simulink model "ISController"  (R2018a)
settings: Solver=FixedStepDiscrete  StartTime=0.0  StopTime=12  FixedStep=0.001  RelTol=1e-3  EnableMultiTasking=on
values from neighbouring files (symbols this model uses):
  Bx_ash_f = 11.7    [ISData.m]    (also in pacjeka_params.m)
  Bx_ash_r = 11.1    [ISData.m]    (also in pacjeka_params.m)
  Bx_snow_f = 10.2    [ISData.m]    (also in pacjeka_params.m)
  Bx_snow_r = 9.71    [ISData.m]    (also in pacjeka_params.m)
  By_ash_f = 8.86    [ISData.m]    (also in pacjeka_params.m)
  By_ash_r = 9.30    (= 9.3)    [ISData.m]    (also in pacjeka_params.m)
  By_snow_f = 19.1    [ISData.m]    (also in pacjeka_params.m)
  By_snow_r = 20.0    (= 20)    [ISData.m]    (also in pacjeka_params.m)
  Cx_ash_f = 1.69    [ISData.m]    (also in pacjeka_params.m)
  Cx_ash_r = 1.69    [ISData.m]    (also in pacjeka_params.m)
  Cx_snow_f = 1.96    [ISData.m]    (also in pacjeka_params.m)
  Cx_snow_r = 1.96    [ISData.m]    (also in pacjeka_params.m)
  Cy_ash_f = 1.19    [ISData.m]    (also in pacjeka_params.m)
  Cy_ash_r = 1.19    [ISData.m]    (also in pacjeka_params.m)
  Cy_snow_f = 0.550    (= 0.55)    [ISData.m]    (also in pacjeka_params.m)
  Cy_snow_r = 0.550    (= 0.55)    [ISData.m]    (also in pacjeka_params.m)
  D_phi = 16000    [ISData.m]    (also in IS_2impulse.m; IS_3impulse.m; IS_4impulse.m; InputShaper.m)
  D_theta = 30960    [ISData.m]    (also in IS_2impulse.m; IS_3impulse.m; IS_4impulse.m; InputShaper.m)
  delta_r = 0    [ISData.m]    (also in IS_2impulse.m; IS_3impulse.m; IS_4impulse.m; InputShaper.m)
  DLCTest = [0 0 0 0 0 0 0 0 0 0 0 0 ... (12003 elements, 12003x1)]    [DLCTest.mat]
  epsilon = 0.4    [ISData.m]    (also in IS_2impulse.m; IS_3impulse.m; IS_4impulse.m; InputShaper.m)
  Ex_ash_f = 0.377    [ISData.m]    (also in pacjeka_params.m)
  Ex_ash_r = 0.362    [ISData.m]    (also in pacjeka_params.m)
  Ex_snow_f = 0.651    [ISData.m]    (also in pacjeka_params.m)
  Ex_snow_r = 0.624    [ISData.m]    (also in pacjeka_params.m)
  Ey_ash_f = -1.21    [ISData.m]    (also in pacjeka_params.m)
  Ey_ash_r = -1.11    [ISData.m]    (also in pacjeka_params.m)
  Ey_snow_f = -2.1    [ISData.m]    (also in pacjeka_params.m)
  Ey_snow_r = -1.93    [ISData.m]    (also in pacjeka_params.m)
  g = 9.81    [ISData.m]    (also in IS_2impulse.m; IS_3impulse.m; IS_4impulse.m; InputShaper.m)
  h = 0.5    [ISData.m]    (also in IS_2impulse.m; IS_3impulse.m; IS_4impulse.m; InputShaper.m)
  Iw = 4    [ISData.m]    (also in IS_2impulse.m; IS_3impulse.m; IS_4impulse.m; InputShaper.m)
  Ixx = 602.1923    [ISData.m]    (also in IS_2impulse.m; IS_3impulse.m; IS_4impulse.m; InputShaper.m)
  Iyy = 2.7370e+03    (= 2737)    [ISData.m]    (also in IS_2impulse.m; IS_3impulse.m; IS_4impulse.m; InputShaper.m)
  Izz = 3070    [ISData.m]    (also in IS_2impulse.m; IS_3impulse.m; IS_4impulse.m; InputShaper.m)
  K_phi = 178000    [ISData.m]    (also in IS_2impulse.m; IS_3impulse.m; IS_4impulse.m; InputShaper.m)
  K_theta = 363540    [ISData.m]    (also in IS_2impulse.m; IS_3impulse.m; IS_4impulse.m; InputShaper.m)
  l_f = 1.2110    (= 1.211)    [ISData.m]    (also in IS_2impulse.m; IS_3impulse.m; IS_4impulse.m; InputShaper.m)
  l_r = 1.4590    (= 1.459)    [ISData.m]    (also in IS_2impulse.m; IS_3impulse.m; IS_4impulse.m; InputShaper.m)
  m = 1830    [ISData.m]    (also in IS_2impulse.m; IS_3impulse.m; IS_4impulse.m; InputShaper.m)
  mu_x_ash_f = 1.20    (= 1.2)    [ISData.m]    (also in pacjeka_params.m)
  mu_x_ash_r = 1.20    (= 1.2)    [ISData.m]    (also in pacjeka_params.m)
  mu_x_snow_f = 0.407    [ISData.m]    (also in pacjeka_params.m)
  mu_x_snow_r = 0.409    [ISData.m]    (also in pacjeka_params.m)
  mu_y_ash_f = 0.935    [ISData.m]    (also in pacjeka_params.m)
  mu_y_ash_r = 0.961    [ISData.m]    (also in pacjeka_params.m)
  mu_y_snow_f = 0.383    [ISData.m]    (also in pacjeka_params.m)
  mu_y_snow_r = 0.394    [ISData.m]    (also in pacjeka_params.m)
  omega0 = Vx0/Rw    (= 64.7813411079)    [ISData.m]    (also in IS_2impulse.m = 74.1; IS_3impulse.m = 74.1; IS_4impulse.m = 74.1; InputShaper.m = 74.0666666667)
  road = 1    [ISData.m]    (also in IS_2impulse.m; IS_3impulse.m; IS_4impulse.m; InputShaper.m)
  Rw = 0.3430    (= 0.343)    [ISData.m]    (also in IS_2impulse.m = 0.3; IS_3impulse.m = 0.3; IS_4impulse.m = 0.3; InputShaper.m = 0.3)
  thetaSW_actual = [thetaSW_actual, deltaSW]    [IS_2impulse.m]    (also in InputShaper.m; InputShaper2.m; thetaSW_IS_L.mat = [0 0 0 0 0 0 0 0 0 0 0 0 ... (12003 elements, 1x12003)]; thetaSW_IS_NL.mat = [0 0 0 0 0 0 0 0 0 0 0 0 ... (12003 elements, 1x12003)])
  Ts = 0.001    [ISData.m]    (also in IS_2impulse.m; IS_3impulse.m; IS_4impulse.m; InputShaper.m)
  Tsmall = 0.001    [ISData.m]    (also in IS_2impulse.m; IS_3impulse.m; IS_4impulse.m; InputShaper.m)
  Vx0 = 22.22    [ISData.m]    (also in IS_2impulse.m = states(3); IS_3impulse.m = states(3); IS_4impulse.m = states(3); InputShaper.m = states(3))
  w = 0.7700    (= 0.77)    [ISData.m]    (also in IS_2impulse.m; IS_3impulse.m; IS_4impulse.m; InputShaper.m)
libraries: simulink x2
(part 2 of 4)

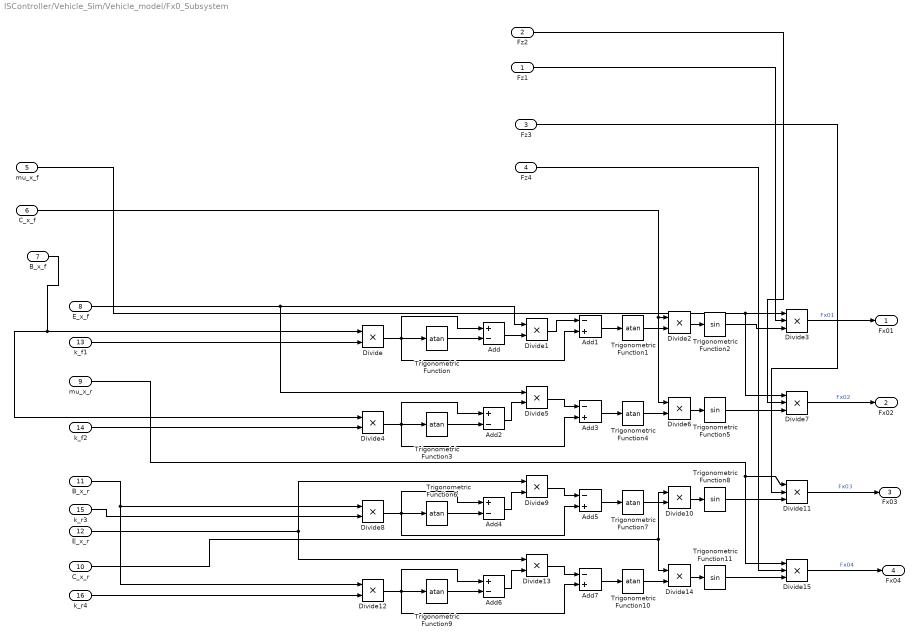
== system ISController/Vehicle_Sim/Vehicle_model/Fx0_Subsystem ==
  Fz1 : Inport  OutDataTypeStr=double  SampleTime=Ts
  Fz2 : Inport  Port=2  OutDataTypeStr=double  SampleTime=Ts
  Fz3 : Inport  Port=3  OutDataTypeStr=double  SampleTime=Ts
  Fz4 : Inport  Port=4  OutDataTypeStr=double  SampleTime=Ts
  mu_x_f : Inport  Port=5
  C_x_f : Inport  Port=6
  B_x_f : Inport  Port=7
  E_x_f : Inport  Port=8
  mu_x_r : Inport  Port=9
  C_x_r : Inport  Port=10
  B_x_r : Inport  Port=11
  E_x_r : Inport  Port=12
  k_f1 : Inport  Port=13
  k_f2 : Inport  Port=14
  k_r3 : Inport  Port=15
  k_r4 : Inport  Port=16
  Add{,2,4,6} (4 alike) : Sum  Inputs=+-
  Add{1,3,5,7} (4 alike) : Sum  Inputs=-+
  Divide{,1..2,4..6,8..10,12..14} (12 alike) : Product  Inputs=**
  Divide{3,7,11,15} (4 alike) : Product  Inputs=***
  Trigonometric Function{,1,3..4,6..7,9..10} (8 alike) : Trigonometry  Operator=atan
  Trigonometric Function{2,5,8,11} (4 alike) : Trigonometry
  Fx01 : Outport  OutDataTypeStr=double  SampleTime=Ts
  Fx02 : Outport  Port=2  OutDataTypeStr=double  SampleTime=Ts
  Fx03 : Outport  Port=3  OutDataTypeStr=double  SampleTime=Ts
  Fx04 : Outport  Port=4  OutDataTypeStr=double  SampleTime=Ts
  wires:
  Divide13/1 -> Add7/1
  Trigonometric Function2/1 -> Divide3/3
  Divide11/1 -> Fx03/1  "Fx03"
  Divide7/1 -> Fx02/1  "Fx02"
  Divide1/1 -> Add1/1
  Trigonometric Function/1 -> Add/2
  Divide15/1 -> Fx04/1  "Fx04"
  Add/1 -> Divide1/2
  Divide/1 -> Add1/2, Add/1, Trigonometric Function/1
  k_f1/1 -> Divide/2
  k_r4/1 -> Divide12/2
  k_r3/1 -> Divide8/2
  Divide6/1 -> Trigonometric Function5/1
  Divide4/1 -> Add3/2, Add2/1, Trigonometric Function3/1
  Divide5/1 -> Add3/1
  Trigonometric Function3/1 -> Add2/2
  Add2/1 -> Divide5/2
  E_x_f/1 -> Divide5/1, Divide1/1
  B_x_f/1 -> Divide4/1, Divide/1
  Trigonometric Function4/1 -> Divide6/2
  C_x_f/1 -> Divide6/1, Divide2/1
  Trigonometric Function5/1 -> Divide7/3
  Add3/1 -> Trigonometric Function4/1
  C_x_r/1 -> Divide14/1, Divide10/1
  B_x_r/1 -> Divide12/1, Divide8/1
  E_x_r/1 -> Divide9/1, Divide13/1
  mu_x_r/1 -> Divide15/1, Divide11/1
  Fz2/1 -> Divide7/2
  mu_x_f/1 -> Divide7/1, Divide3/1
  k_f2/1 -> Divide4/2
  Fz1/1 -> Divide3/2
  Fz3/1 -> Divide11/2
  Add1/1 -> Trigonometric Function1/1
  Add4/1 -> Divide9/2
  Divide8/1 -> Add5/2, Add4/1, Trigonometric Function6/1
  Trigonometric Function8/1 -> Divide11/3
  Add5/1 -> Trigonometric Function7/1
  Trigonometric Function6/1 -> Add4/2
  Divide10/1 -> Trigonometric Function8/1
  Trigonometric Function7/1 -> Divide10/2
  Fz4/1 -> Divide15/2
  Divide9/1 -> Add5/1
  Trigonometric Function1/1 -> Divide2/2
  Divide3/1 -> Fx01/1  "Fx01"
  Divide2/1 -> Trigonometric Function2/1
  Trigonometric Function10/1 -> Divide14/2
  Trigonometric Function9/1 -> Add6/2
  Divide14/1 -> Trigonometric Function11/1
  Divide12/1 -> Add7/2, Add6/1, Trigonometric Function9/1
  Trigonometric Function11/1 -> Divide15/3
  Add7/1 -> Trigonometric Function10/1
  Add6/1 -> Divide13/2

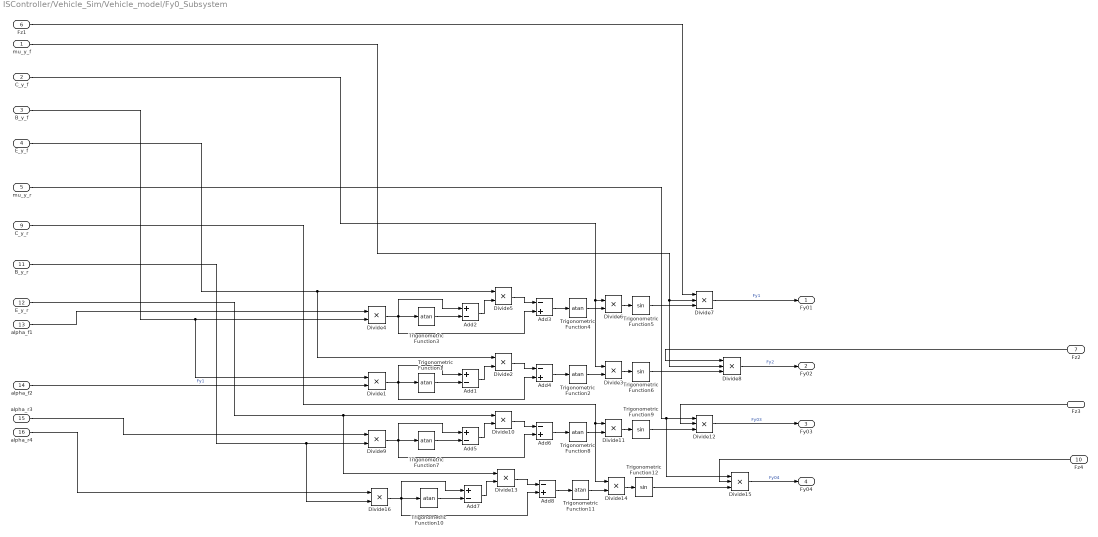
== system ISController/Vehicle_Sim/Vehicle_model/Fy0_Subsystem ==
  mu_y_f : Inport  OutDataTypeStr=double  SampleTime=Ts
  C_y_f : Inport  Port=2  OutDataTypeStr=double  SampleTime=Ts
  B_y_f : Inport  Port=3  OutDataTypeStr=double  SampleTime=Ts
  E_y_f : Inport  Port=4  OutDataTypeStr=double  SampleTime=Ts
  mu_y_r : Inport  Port=5  OutDataTypeStr=double  SampleTime=Ts
  Fz1 : Inport  Port=6  OutDataTypeStr=double  SampleTime=Ts
  Fz2 : Inport  Port=7  OutDataTypeStr=double  SampleTime=Ts
  Fz3 : Inport  Port=8  OutDataTypeStr=double  SampleTime=Ts
  C_y_r : Inport  Port=9  OutDataTypeStr=double  SampleTime=Ts
  Fz4 : Inport  Port=10  OutDataTypeStr=double  SampleTime=Ts
  B_y_r : Inport  Port=11  OutDataTypeStr=double  SampleTime=Ts
  E_y_r : Inport  Port=12  OutDataTypeStr=double  SampleTime=Ts
  alpha_f1 : Inport  Port=13  OutDataTypeStr=double  SampleTime=Ts
  alpha_f2 : Inport  Port=14  OutDataTypeStr=double  SampleTime=Ts
  alpha_r3 : Inport  Port=15  OutDataTypeStr=double  SampleTime=Ts
  alpha_r4 : Inport  Port=16  OutDataTypeStr=double  SampleTime=Ts
  Add{1..2,5,7} (4 alike) : Sum  Inputs=+-
  Add{3..4,6,8} (4 alike) : Sum  Inputs=-+
  Divide{1..6,9..11,13..14,16} (12 alike) : Product  Inputs=**
  Divide{7..8,12,15} (4 alike) : Product  Inputs=***
  Trigonometric Function{1..4,7..8,10..11} (8 alike) : Trigonometry  Operator=atan
  Trigonometric Function{5..6,9,12} (4 alike) : Trigonometry
  Fy01 : Outport  OutDataTypeStr=double  SampleTime=Ts
  Fy02 : Outport  Port=2  OutDataTypeStr=double  SampleTime=Ts
  Fy03 : Outport  Port=3  OutDataTypeStr=double  SampleTime=Ts
  Fy04 : Outport  Port=4  OutDataTypeStr=double  SampleTime=Ts
  wires:
  Add6/1 -> Trigonometric Function8/1
  Trigonometric Function9/1 -> Divide12/3
  alpha_r3/1 -> Divide9/1
  alpha_r4/1 -> Divide16/1
  C_y_f/1 -> Divide6/1, Divide3/1
  B_y_f/1 -> Divide4/2, Divide1/1
  alpha_f1/1 -> Divide4/1
  E_y_r/1 -> Divide13/1, Divide10/1
  B_y_r/1 -> Divide16/2, Divide9/2
  mu_y_r/1 -> Divide12/1, Divide15/1
  E_y_f/1 -> Divide5/1, Divide2/1
  mu_y_f/1 -> Divide8/2, Divide7/2
  Trigonometric Function1/1 -> Add1/2
  Add1/1 -> Divide2/2
  Trigonometric Function6/1 -> Divide8/3
  Trigonometric Function2/1 -> Divide3/2
  Divide1/1 -> Add4/2, Add1/1, Trigonometric Function1/1
  Divide3/1 -> Trigonometric Function6/1
  Divide2/1 -> Add4/1
  Add4/1 -> Trigonometric Function2/1
  Fz4/1 -> Divide15/2
  Fz3/1 -> Divide12/2
  Fz2/1 -> Divide8/1
  Fz1/1 -> Divide7/1
  C_y_r/1 -> Divide14/1, Divide11/1
  Divide15/1 -> Fy04/1  "Fy04"
  Trigonometric Function12/1 -> Divide15/3
  Add8/1 -> Trigonometric Function11/1
  Divide16/1 -> Add8/2, Add7/1, Trigonometric Function10/1
  Trigonometric Function11/1 -> Divide14/2
  Add7/1 -> Divide13/2
  Divide13/1 -> Add8/1
  Divide14/1 -> Trigonometric Function12/1
  Trigonometric Function10/1 -> Add7/2
  Divide12/1 -> Fy03/1  "Fy03"
  Divide9/1 -> Add6/2, Add5/1, Trigonometric Function7/1
  Trigonometric Function7/1 -> Add5/2
  Add5/1 -> Divide10/2
  Trigonometric Function5/1 -> Divide7/3
  Divide11/1 -> Trigonometric Function9/1
  Divide6/1 -> Trigonometric Function5/1
  Add3/1 -> Trigonometric Function4/1
  Trigonometric Function3/1 -> Add2/2
  Divide10/1 -> Add6/1
  Add2/1 -> Divide5/2
  Trigonometric Function4/1 -> Divide6/2
  Divide4/1 -> Add3/2, Add2/1, Trigonometric Function3/1
  Divide5/1 -> Add3/1
  Trigonometric Function8/1 -> Divide11/2
  Divide7/1 -> Fy01/1  "Fy1"
  Divide8/1 -> Fy02/1  "Fy2"
  alpha_f2/1 -> Divide1/2  "Fy1"

== system ISController/Vehicle_Sim/Vehicle_model/Fy0_to_Fy_subsystem ==
  mu_x_f : Inport  OutDataTypeStr=double  SampleTime=Ts
  mu_x_r : Inport  Port=2  OutDataTypeStr=double  SampleTime=Ts
  Fx01 : Inport  Port=3  OutDataTypeStr=double  SampleTime=Ts
  Fx02 : Inport  Port=4  OutDataTypeStr=double  SampleTime=Ts
  Fx03 : Inport  Port=5  OutDataTypeStr=double  SampleTime=Ts
  Fx04 : Inport  Port=6  OutDataTypeStr=double  SampleTime=Ts
  Fz1 : Inport  Port=7  OutDataTypeStr=double  SampleTime=Ts
  Fz2 : Inport  Port=8  OutDataTypeStr=double  SampleTime=Ts
  Fz3 : Inport  Port=9  OutDataTypeStr=double  SampleTime=Ts
  Fz4 : Inport  Port=10  OutDataTypeStr=double  SampleTime=Ts
  Fy01 : Inport  Port=11  OutDataTypeStr=double  SampleTime=Ts
  Fy02 : Inport  Port=12  OutDataTypeStr=double  SampleTime=Ts
  Fy03 : Inport  Port=13  OutDataTypeStr=double  SampleTime=Ts
  Fy04 : Inport  Port=14  OutDataTypeStr=double  SampleTime=Ts
  Add{,1..3} (4 alike) : Sum  Inputs=+-
  Constant{,1..3} (4 alike) : Constant
  Divide{,3,6,9} (4 alike) : Product  Inputs=*/
  Divide{1..2,4..5,7..8,10..11} (8 alike) : Product  Inputs=**
  Sqrt{,1..3} (4 alike) : Sqrt  SaturateOnIntegerOverflow=on
  Square{,1..3} (4 alike) : Math  Operator=square  RndMeth=Zero  SaturateOnIntegerOverflow=on
  local_Fy1 : Outport  OutDataTypeStr=double  SampleTime=Ts
  local_Fy2 : Outport  Port=2  OutDataTypeStr=double  SampleTime=Ts
  local_Fy3 : Outport  Port=3  OutDataTypeStr=double  SampleTime=Ts
  lcoal_Fy4 : Outport  Port=4  OutDataTypeStr=double  SampleTime=Ts
  wires:
  Divide1/1 -> Divide/2
  Divide/1 -> Square/1
  Constant/1 -> Add/1
  Divide2/1 -> local_Fy1/1  "Fy1"
  Divide11/1 -> lcoal_Fy4/1  "Fy4"
  Fz4/1 -> Divide10/2  "Fz4"
  mu_x_f/1 -> Divide4/1, Divide1/1  "mu_x_f"
  Fx04/1 -> Divide9/1  "Fx04"
  Fx01/1 -> Divide/1  "Fx01"
  Fz3/1 -> Divide7/2  "Fz3"
  Fx02/1 -> Divide3/1  "Fx02"
  mu_x_r/1 -> Divide10/1, Divide7/1  "mu_x_r"
  Fx03/1 -> Divide6/1  "Fx03"
  Fz1/1 -> Divide1/2  "Fz1"
  Fz2/1 -> Divide4/2  "Fz2"
  Square2/1 -> Add2/2
  Divide6/1 -> Square2/1
  Sqrt2/1 -> Divide8/1
  Constant2/1 -> Add2/1
  Sqrt3/1 -> Divide11/1
  Constant3/1 -> Add3/1
  Add3/1 -> Sqrt3/1
  Divide9/1 -> Square3/1
  Square3/1 -> Add3/2
  Add/1 -> Sqrt/1
  Square/1 -> Add/2
  Divide10/1 -> Divide9/2
  Divide8/1 -> local_Fy3/1  "Fy3"
  Sqrt/1 -> Divide2/1
  Divide4/1 -> Divide3/2
  Square1/1 -> Add1/2
  Divide3/1 -> Square1/1
  Constant1/1 -> Add1/1
  Fy02/1 -> Divide5/2  "Fy02"
  Add1/1 -> Sqrt1/1
  Sqrt1/1 -> Divide5/1
  Divide7/1 -> Divide6/2
  Add2/1 -> Sqrt2/1
  Fy03/1 -> Divide8/2  "Fy03"
  Divide5/1 -> local_Fy2/1  "Fy2"
  Fy01/1 -> Divide2/2  "Fy01"
  Fy04/1 -> Divide11/2  "Fy04"

== system ISController/Vehicle_Sim/Vehicle_model/Fz_Subsystem ==
  l_f : Inport  OutDataTypeStr=double  SampleTime=Ts
  l_r : Inport  Port=2  OutDataTypeStr=double  SampleTime=Ts
  k_phi : Inport  Port=3  OutDataTypeStr=double  SampleTime=Ts
  d_phi : Inport  Port=4  OutDataTypeStr=double  SampleTime=Ts
  theta_dot : Inport  Port=5  OutDataTypeStr=double  SampleTime=Ts
  theta : Inport  Port=6  OutDataTypeStr=double  SampleTime=Ts
  phi_dot : Inport  Port=7  OutDataTypeStr=double  SampleTime=Ts
  phi : Inport  Port=8  OutDataTypeStr=double  SampleTime=Ts
  K_theta : Inport  Port=9  OutDataTypeStr=double  SampleTime=Ts
  D_theta : Inport  Port=10  OutDataTypeStr=double  SampleTime=Ts
  w : Inport  Port=11  OutDataTypeStr=double  SampleTime=Ts
  Add{,1,3..4,6} (5 alike) : Sum
  Add2 : Sum  Inputs=+-+
  Add5 : Sum  Inputs=--
  Add7 : Sum  Inputs=-+
  Add8 : Sum  Inputs=-+
  Divide{,1..2,5} (4 alike) : Product  Inputs=*/
  Divide3 : Product  Inputs=**
  Divide4 : Product  Inputs=**
  Gain : Gain  Gain=-1  OutDataTypeStr=double
  Gain1 : Gain  Gain=0.5
  mg : Constant  Value=m*g
  tau_phi_subsystem : Subsystem
  tau_theta_subsystem : Subsystem
  Fz1 : Outport  OutDataTypeStr=double  SampleTime=Ts
  Fz2 : Outport  Port=2  OutDataTypeStr=double  SampleTime=Ts
  Fz3 : Outport  Port=3  OutDataTypeStr=double  SampleTime=Ts
  Fz4 : Outport  Port=4  OutDataTypeStr=double  SampleTime=Ts
  wires:
  phi/1 -> tau_phi_subsystem/4(phi)
  theta/1 -> tau_theta_subsystem/2(theta)
  phi_dot/1 -> tau_phi_subsystem/3(phi_dot)
  w/1 -> Divide2/2, Gain/1
  Add1/1 -> Divide2/1
  Divide2/1 -> Add3/1
  Add2/1 -> Divide5/1
  d_phi/1 -> tau_phi_subsystem/2(D_phi)
  D_theta/1 -> tau_theta_subsystem/4(D_theta)
  l_r/1 -> Divide4/1, Add5/1
  theta_dot/1 -> tau_theta_subsystem/1(theta_dot)
  tau_theta_subsystem/1(tau_theta) -> Add2/1  "tau_theta"
  K_theta/1 -> tau_theta_subsystem/3(K_theta)
  Add8/1 -> Fz1/1  "Fz1"
  Add/1 -> Add8/2, Add4/1  "E1"
  Divide3/1 -> Add2/2
  Divide5/1 -> Fz4/1, Add8/1, Add7/1, Add6/1  "Fz4"
  Add3/1 -> Gain1/1
  Add5/1 -> Divide5/2
  Gain1/1 -> Add7/2, Add4/2, Add/2  "E2"
  Add4/1 -> Divide3/2
  Add6/1 -> Fz3/1  "Fz3"
  Divide/1 -> Divide4/2, Add6/2  "E3"
  mg/1 -> Add3/2
  Divide4/1 -> Add2/3
  Divide1/1 -> Add/1
  k_phi/1 -> tau_phi_subsystem/1(K_phi)
  l_f/1 -> Add5/2, Divide3/1
  Add7/1 -> Fz2/1  "Fz2"
  tau_phi_subsystem/1(tau_phi_f) -> Divide1/1, Add1/1  "tau_phi_f"
  tau_phi_subsystem/2(tau_phi_r) -> Add1/2, Divide/1  "tau_phi_r"
  Gain/1 -> Divide1/2, Divide/2

== system ISController/Vehicle_Sim/Vehicle_model/Pacjeka_parameters_Subsystem ==
  surface_condition : Inport  OutDataTypeStr=double  SampleTime=Ts
  Ashphalt_condition_subsystem : Subsystem  TreatAsAtomicUnit=on
  Demux : Demux  Outputs=2
  If : If  IfExpression=(u1==1)
  Merge : Merge
  Snow_condition_subsystem : Subsystem  TreatAsAtomicUnit=on
  front : Outport  OutDataTypeStr=double  SampleTime=Ts
  rear : Outport  Port=2  OutDataTypeStr=double  SampleTime=Ts
  wires:
  Demux/2 -> rear/1  "rear"
  Merge/1 -> Demux/1
  If/1 -> Ashphalt_condition_subsystem/Action
  If/2 -> Snow_condition_subsystem/Action
  Demux/1 -> front/1  "front"
  surface_condition/1 -> If/1
  Ashphalt_condition_subsystem/1(Out1) -> Merge/1
  Snow_condition_subsystem/1(Out1) -> Merge/2

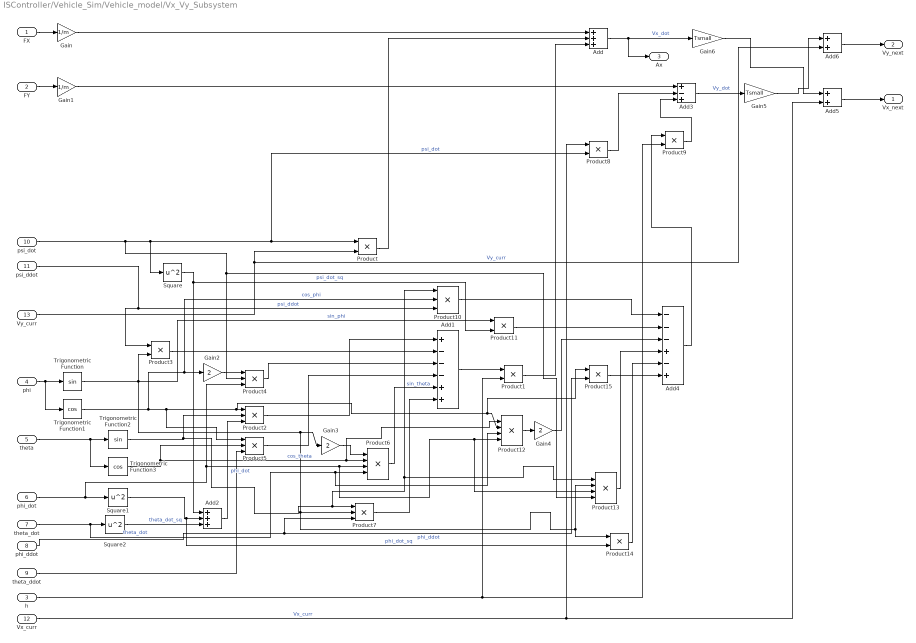
== system ISController/Vehicle_Sim/Vehicle_model/Vx_Vy_Subsystem ==
  FX : Inport  OutDataTypeStr=double  SampleTime=Ts
  FY : Inport  Port=2  OutDataTypeStr=double  SampleTime=Ts
  h : Inport  Port=3  OutDataTypeStr=double  SampleTime=Ts
  phi : Inport  Port=4  OutDataTypeStr=double  SampleTime=Ts
  theta : Inport  Port=5  OutDataTypeStr=double  SampleTime=Ts
  phi_dot : Inport  Port=6  OutDataTypeStr=double  SampleTime=Ts
  theta_dot : Inport  Port=7  OutDataTypeStr=double  SampleTime=Ts
  phi_ddot : Inport  Port=8  OutDataTypeStr=double  SampleTime=Ts
  theta_ddot : Inport  Port=9  OutDataTypeStr=double  SampleTime=Ts
  psi_dot : Inport  Port=10  OutDataTypeStr=double  SampleTime=Ts
  psi_ddot : Inport  Port=11  OutDataTypeStr=double  SampleTime=Ts
  Vx_curr : Inport  Port=12  OutDataTypeStr=double  SampleTime=Tsmall
  Vy_curr : Inport  Port=13  OutDataTypeStr=double  SampleTime=Tsmall
  Add : Sum  Inputs=+++
  Add1 : Sum  Inputs=+---++
  Add2 : Sum  Inputs=+++
  Add3 : Sum  Inputs=+-+
  Add4 : Sum  Inputs=---+-+
  Add5 : Sum
  Add6 : Sum
  Gain : Gain  Gain=1/m
  Gain1 : Gain  Gain=1/m
  Gain2 : Gain  Gain=2
  Gain3 : Gain  Gain=2
  Gain4 : Gain  Gain=2
  Gain5 : Gain  Gain=Tsmall
  Gain6 : Gain  Gain=Tsmall
  Product{,1,3,8..9,11,14..15} (8 alike) : Product
  Product{2,4..5,7,10} (5 alike) : Product  Inputs=3
  Product12 : Product  Inputs=4
  Product13 : Product  Inputs=4
  Product6 : Product  Inputs=4
  Square : Math  Operator=square  RndMeth=Zero  SaturateOnIntegerOverflow=on
  Square1 : Math  Operator=square  RndMeth=Zero  SaturateOnIntegerOverflow=on
  Square2 : Math  Operator=square  RndMeth=Zero  SaturateOnIntegerOverflow=on
  Trigonometric Function : Trigonometry
  Trigonometric Function1 : Trigonometry  Operator=cos
  Trigonometric Function2 : Trigonometry
  Trigonometric Function3 : Trigonometry  Operator=cos
  Vx_next : Outport  OutDataTypeStr=double  SampleTime=Tsmall
  Vy_next : Outport  Port=2  OutDataTypeStr=double  SampleTime=Tsmall
  Ax : Outport  Port=3
  wires:
  FX/1 -> Gain/1
  FY/1 -> Gain1/1
  Gain/1 -> Add/1
  psi_dot/1 -> Product4/2, Product13/4, Square/1, Product8/2, Product/1  "psi_dot"
  Product/1 -> Add/2
  Vy_curr/1 -> Add6/2, Product/2  "Vy_curr"
  Product1/1 -> Add/3
  phi/1 -> Trigonometric Function1/1, Trigonometric Function/1
  theta/1 -> Trigonometric Function3/1, Trigonometric Function2/1
  Add1/1 -> Product1/1
  h/1 -> Product9/2, Product1/2
  Add2/1 -> Product2/3
  Square/1 -> Product11/2, Add2/1  "psi_dot_sq"
  Square1/1 -> Product14/2, Add2/2  "phi_dot_sq"
  phi_dot/1 -> Product13/3, Product12/4, Product6/3, Product4/3, Square1/1  "phi_dot"
  Square2/1 -> Add2/3  "theta_dot_sq"
  theta_dot/1 -> Product12/3, Product6/4, Square2/1  "theta_dot"
  Product2/1 -> Add1/1
  Trigonometric Function/1 -> Product11/1, Product14/1, Product13/2, Product7/2, Gain3/1, Product3/2  "sin_phi"
  psi_ddot/1 -> Product10/3, Product3/1  "psi_ddot"
  Product3/1 -> Add1/2
  Gain2/1 -> Product4/1
  Product4/1 -> Add1/3
  Trigonometric Function3/1 -> Product5/2, Product12/1, Product6/2  "cos_theta"
  theta_ddot/1 -> Product5/3
  Product5/1 -> Add1/4
  Product6/1 -> Add1/5
  Gain3/1 -> Product6/1
  phi_ddot/1 -> Product15/2, Product7/3  "phi_ddot"
  Product7/1 -> Add1/6
  Add/1 -> Ax/1, Gain6/1  "Vx_dot"
  Gain1/1 -> Add3/1
  Vx_curr/1 -> Add5/2, Product8/1  "Vx_curr"
  Product8/1 -> Add3/2
  Add4/1 -> Product9/1
  Product9/1 -> Add3/3
  Product10/1 -> Add4/1
  Trigonometric Function2/1 -> Product13/1, Product10/1, Product7/1, Product2/2  "sin_theta"
  Trigonometric Function1/1 -> Product10/2, Gain2/1, Product5/1, Product15/1, Product12/2, Product2/1  "cos_phi"
  Product11/1 -> Add4/2
  Product12/1 -> Gain4/1
  Gain4/1 -> Add4/3
  Product13/1 -> Add4/4
  Product14/1 -> Add4/5
  Product15/1 -> Add4/6
  Add3/1 -> Gain5/1  "Vy_dot"
  Gain5/1 -> Add6/1
  Add5/1 -> Vx_next/1
  Gain6/1 -> Add5/1
  Add6/1 -> Vy_next/1

== system ISController/Vehicle_Sim/Vehicle_model/local_to_global_Fx_Fy_Subsystem ==
  local_Fx1 : Inport  OutDataTypeStr=double  SampleTime=Ts
  local_Fx2 : Inport  Port=2  OutDataTypeStr=double  SampleTime=Ts
  local_Fx3 : Inport  Port=3  OutDataTypeStr=double  SampleTime=Ts
  local_Fx4 : Inport  Port=4  OutDataTypeStr=double  SampleTime=Ts
  local_Fy1 : Inport  Port=5  OutDataTypeStr=double  SampleTime=Ts
  local_Fy2 : Inport  Port=6  OutDataTypeStr=double  SampleTime=Ts
  local_Fy3 : Inport  Port=7  OutDataTypeStr=double  SampleTime=Ts
  local_Fy4 : Inport  Port=8  OutDataTypeStr=double  SampleTime=Ts
  delta_f2 : Inport  Port=9  OutDataTypeStr=double  SampleTime=Ts
  Add{,1..3} (4 alike) : Sum
  Constant : Constant  Value=delta_r
  Cos : Trigonometry  Operator=cos
  Cos1 : Trigonometry  Operator=cos
  Product{,1..15} (16 alike) : Product
  Sin : Trigonometry
  Sin1 : Trigonometry
  Subtract{,1..3} (4 alike) : Sum  Inputs=+-
  Fx1 : Outport  OutDataTypeStr=double  SampleTime=Ts
  Fx2 : Outport  Port=2  OutDataTypeStr=double  SampleTime=Ts
  Fx3 : Outport  Port=3  OutDataTypeStr=double  SampleTime=Ts
  Fx4 : Outport  Port=4  OutDataTypeStr=double  SampleTime=Ts
  Fy1 : Outport  Port=5  OutDataTypeStr=double  SampleTime=Ts
  Fy2 : Outport  Port=6  OutDataTypeStr=double  SampleTime=Ts
  Fy3 : Outport  Port=7  OutDataTypeStr=double  SampleTime=Ts
  Fy4 : Outport  Port=8  OutDataTypeStr=double  SampleTime=Ts
  wires:
  delta_f2/1 -> Cos/1, Sin/1
  local_Fx1/1 -> Product2/2, Product/1  "local_Fx1"
  local_Fx2/1 -> Product6/2, Product4/2  "local_Fx2"
  local_Fx3/1 -> Product10/2, Product8/1  "local_Fx3"
  local_Fx4/1 -> Product14/1, Product12/1  "local_Fx4"
  local_Fy1/1 -> Product3/2, Product1/1  "local_Fy1"
  local_Fy2/1 -> Product7/2, Product5/2  "local_Fy2"
  local_Fy3/1 -> Product11/2, Product9/2  "local_Fy3"
  local_Fy4/1 -> Product15/1, Product13/1  "local_Fy4"
  Cos/1 -> Product7/1, Product4/1, Product3/1, Product/2  "cosDeltaf2"
  Sin/1 -> Product5/1, Product6/1, Product2/1, Product1/2  "sinDeltaf2"
  Product/1 -> Subtract/1
  Product1/1 -> Subtract/2
  Subtract/1 -> Fx1/1  "Fx1"
  Product2/1 -> Add/1
  Product3/1 -> Add/2
  Add/1 -> Fy1/1  "Fy1"
  Product6/1 -> Add1/1
  Product7/1 -> Add1/2
  Product4/1 -> Subtract1/1
  Product5/1 -> Subtract1/2
  Subtract1/1 -> Fx2/1  "Fx2"
  Add1/1 -> Fy2/1  "Fy2"
  Constant/1 -> Cos1/1, Sin1/1
  Sin1/1 -> Product14/2, Product13/2, Product10/1, Product9/1  "sinDelta_r"
  Cos1/1 -> Product15/2, Product12/2, Product11/1, Product8/2  "cosDelta_r"
  Product8/1 -> Subtract2/1
  Product9/1 -> Subtract2/2
  Subtract2/1 -> Fx3/1  "Fx3"
  Product10/1 -> Add2/1
  Product11/1 -> Add2/2
  Add2/1 -> Fy3/1  "Fy3"
  Product12/1 -> Subtract3/1
  Product13/1 -> Subtract3/2
  Product14/1 -> Add3/1
  Product15/1 -> Add3/2
  Subtract3/1 -> Fx4/1  "Fx4"
  Add3/1 -> Fy4/1  "Fy4"

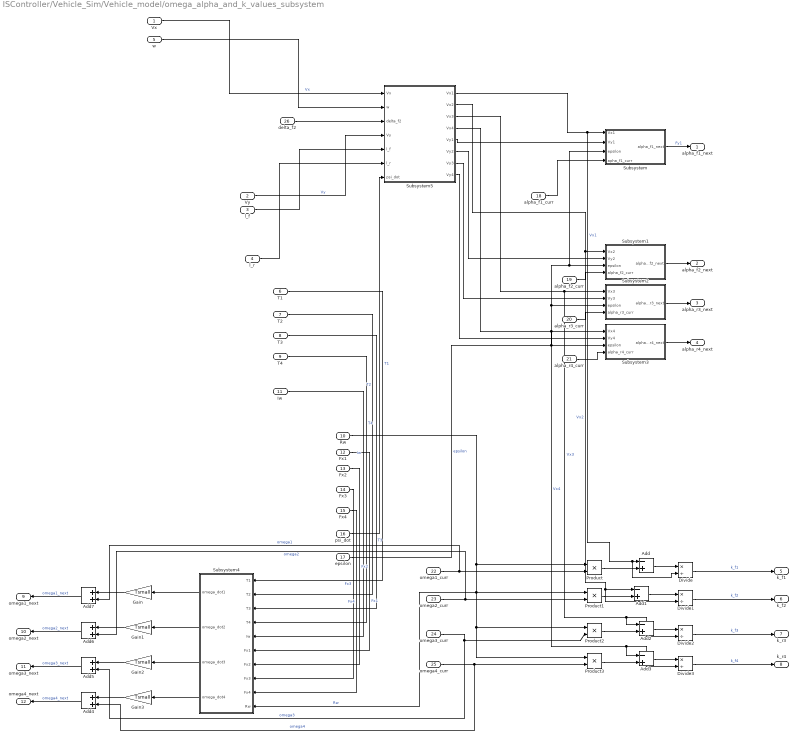
== system ISController/Vehicle_Sim/Vehicle_model/omega_alpha_and_k_values_subsystem ==
  Vx : Inport  OutDataTypeStr=double  SampleTime=Ts
  Vy : Inport  Port=2  OutDataTypeStr=double  SampleTime=Ts
  l_f : Inport  Port=3  OutDataTypeStr=double  SampleTime=Ts
  l_r : Inport  Port=4  OutDataTypeStr=double  SampleTime=Ts
  w : Inport  Port=5  OutDataTypeStr=double  SampleTime=Ts
  T1 : Inport  Port=6  OutDataTypeStr=double  SampleTime=Ts
  T2 : Inport  Port=7  OutDataTypeStr=double  SampleTime=Ts
  T3 : Inport  Port=8  OutDataTypeStr=double  SampleTime=Ts
  T4 : Inport  Port=9  OutDataTypeStr=double  SampleTime=Ts
  Rw : Inport  Port=10  OutDataTypeStr=double  SampleTime=Ts
  Iw : Inport  Port=11  OutDataTypeStr=double  SampleTime=Ts
  Fx1 : Inport  Port=12  OutDataTypeStr=double  SampleTime=Ts
  Fx2 : Inport  Port=13  OutDataTypeStr=double  SampleTime=Ts
  Fx3 : Inport  Port=14  OutDataTypeStr=double  SampleTime=Ts
  Fx4 : Inport  Port=15  OutDataTypeStr=double  SampleTime=Ts
  psi_dot : Inport  Port=16  OutDataTypeStr=double  SampleTime=Ts
  epsilon : Inport  Port=17  OutDataTypeStr=double  SampleTime=Ts
  alpha_f1_curr : Inport  Port=18  OutDataTypeStr=double  SampleTime=Tsmall
  alpha_f2_curr : Inport  Port=19  OutDataTypeStr=double  SampleTime=Tsmall
  alpha_r3_curr : Inport  Port=20  OutDataTypeStr=double  SampleTime=Tsmall
  alpha_r4_curr : Inport  Port=21  OutDataTypeStr=double  SampleTime=Tsmall
  omega1_curr : Inport  Port=22  OutDataTypeStr=double  SampleTime=Ts
  omega2_curr : Inport  Port=23  OutDataTypeStr=double  SampleTime=Ts
  omega3_curr : Inport  Port=24  OutDataTypeStr=double  SampleTime=Ts
  omega4_curr : Inport  Port=25  OutDataTypeStr=double  SampleTime=Ts
  delta_f2 : Inport  Port=26  OutDataTypeStr=double  SampleTime=Ts
  Add{,1..3} (4 alike) : Sum  Inputs=-+
  Add{4..7} (4 alike) : Sum
  Divide{,1..3} (4 alike) : Product  Inputs=*/
  Gain{,1..3} (4 alike) : Gain  Gain=Tsmall
  Product{,1..3} (4 alike) : Product
  Subsystem : Subsystem
  Subsystem1 : Subsystem
  Subsystem2 : Subsystem
  Subsystem3 : Subsystem
  Subsystem4 : Subsystem
  Subsystem5 : Subsystem
  alpha_f1_next : Outport  OutDataTypeStr=double  SampleTime=Ts
  alpha_f2_next : Outport  Port=2  OutDataTypeStr=double  SampleTime=Tsmall
  alpha_r3_next : Outport  Port=3  OutDataTypeStr=double  SampleTime=Tsmall
  alpha_r4_next : Outport  Port=4  OutDataTypeStr=double  SampleTime=Tsmall
  k_f1 : Outport  Port=5  OutDataTypeStr=double  SampleTime=Ts
  k_f2 : Outport  Port=6  OutDataTypeStr=double  SampleTime=Ts
  k_r3 : Outport  Port=7  OutDataTypeStr=double  SampleTime=Ts
  k_r4 : Outport  Port=8  OutDataTypeStr=double  SampleTime=Ts
  omega1_next : Outport  Port=9
  omega2_next : Outport  Port=10
  omega3_next : Outport  Port=11
  omega4_next : Outport  Port=12
  wires:
  Subsystem5/1(Vx1) -> Divide/2, Add/1, Subsystem/1(Vx1)  "Vx1"
  epsilon/1 -> Subsystem3/3(epsilon), Subsystem2/3(epsilon), Subsystem1/3(epsilon), Subsystem/3(epsilon)  "epsilon"
  Subsystem1/1(alpha_f2_next) -> alpha_f2_next/1
  Divide/1 -> k_f1/1  "k_f1"
  omega1_curr/1 -> Add7/2, Product/2  "omega1"
  omega2_curr/1 -> Add6/2, Product1/2  "omega2"
  omega3_curr/1 -> Add5/2, Product2/2  "omega3"
  omega4_curr/1 -> Add4/2, Product3/2  "omega4"
  Rw/1 -> Subsystem4/10(Rw), Product1/1, Product3/1, Product2/1, Product/1  "Rw"
  Product/1 -> Add/2
  Add/1 -> Divide/1
  Product1/1 -> Add1/2
  Add1/1 -> Divide1/1
  Product2/1 -> Add2/2
  Add2/1 -> Divide2/1
  Product3/1 -> Add3/2
  Add3/1 -> Divide3/1
  Divide1/1 -> k_f2/1  "k_f2"
  Divide2/1 -> k_r3/1  "k_f3"
  Divide3/1 -> k_r4/1  "k_f4"
  T1/1 -> Subsystem4/1(T1)  "T1"
  T2/1 -> Subsystem4/2(T2)  "T2"
  T3/1 -> Subsystem4/3(T3)  "T3"
  T4/1 -> Subsystem4/4(T4)  "T4"
  Iw/1 -> Subsystem4/5(Iw)  "Iw"
  Fx1/1 -> Subsystem4/6(Fx1)  "Fx1"
  Fx2/1 -> Subsystem4/7(Fx2)  "Fx2"
  Fx3/1 -> Subsystem4/8(Fx3)  "Fx3"
  Fx4/1 -> Subsystem4/9(Fx4)  "Fx4"
  Subsystem4/1(omega_dot1) -> Gain/1
  Subsystem4/2(omega_dot2) -> Gain1/1
  Subsystem4/3(omega_dot3) -> Gain2/1
  Subsystem4/4(omega_dot4) -> Gain3/1
  alpha_f1_curr/1 -> Subsystem/4(apha_f1_curr)
  alpha_f2_curr/1 -> Subsystem1/4(alpha_f2_curr)
  Subsystem2/1(alpha_r3_next) -> alpha_r3_next/1
  alpha_r3_curr/1 -> Subsystem2/4(alpha_r3_curr)
  Subsystem3/1(alpha_r4_next) -> alpha_r4_next/1
  alpha_r4_curr/1 -> Subsystem3/4(alpha_r4_curr)
  Gain1/1 -> Add6/1
  Gain/1 -> Add7/1
  Gain2/1 -> Add5/1
  Gain3/1 -> Add4/1
  Add7/1 -> omega1_next/1  "omega1_next"
  Add6/1 -> omega2_next/1  "omega2_next"
  Add5/1 -> omega3_next/1  "omega3_next"
  Add4/1 -> omega4_next/1  "omega4_next"
  Subsystem5/2(Vx2) -> Divide1/2, Add1/1, Subsystem1/1(Vx2)  "Vx2"
  Subsystem5/4(Vx4) -> Subsystem3/1(Vx4), Add3/1, Divide3/2  "Vx4"
  Subsystem5/3(Vx3) -> Subsystem2/1(Vx3), Add2/1, Divide2/2  "Vx3"
  Vx/1 -> Subsystem5/1(Vx)  "Vx"
  w/1 -> Subsystem5/2(w)
  Vy/1 -> Subsystem5/4(Vy)  "Vy"
  l_f/1 -> Subsystem5/5(l_f)
  l_r/1 -> Subsystem5/6(l_r)
  psi_dot/1 -> Subsystem5/7(psi_dot)
  Subsystem5/5(Vy1) -> Subsystem/2(Vy1)
  Subsystem5/6(Vy2) -> Subsystem1/2(Vy2)
  Subsystem5/7(Vy3) -> Subsystem2/2(Vy3)
  Subsystem5/8(Vy4) -> Subsystem3/2(Vy4)
  delta_f2/1 -> Subsystem5/3(delta_f2)
  Subsystem/1(alpha_f1_next) -> alpha_f1_next/1  "Fy1"

== system ISController/Vehicle_Sim/Vehicle_model/phi_subsystem ==
  FY : Inport  OutDataTypeStr=double  SampleTime=Ts
  psi_dot : Inport  Port=2  OutDataTypeStr=double  SampleTime=Tsmall
  phi_dot : Inport  Port=3  OutDataTypeStr=double  SampleTime=Tsmall
  phi : Inport  Port=4  OutDataTypeStr=double  SampleTime=Tsmall
  theta_dot : Inport  Port=5  OutDataTypeStr=double  SampleTime=Tsmall
  theta : Inport  Port=6  OutDataTypeStr=double  SampleTime=Tsmall
  Ixx : Inport  Port=7  OutDataTypeStr=double  SampleTime=Ts
  Iyy : Inport  Port=8  OutDataTypeStr=double  SampleTime=Ts
  Izz : Inport  Port=9  OutDataTypeStr=double  SampleTime=Ts
  K_phi : Inport  Port=10  OutDataTypeStr=double  SampleTime=Ts
  D_phi : Inport  Port=11  OutDataTypeStr=double  SampleTime=Ts
  h : Inport  Port=12  OutDataTypeStr=double  SampleTime=Ts
  Divide : Product  Inputs=*/
  phi_ddot_denominator_subsystem : Subsystem
  phi_ddot_numerator_subsystem : Subsystem
  phi_ddot : Outport  OutDataTypeStr=double  SampleTime=Tsmall
  wires:
  phi_ddot_numerator_subsystem/1(phi_ddot_numerator) -> Divide/1
  phi/1 -> phi_ddot_denominator_subsystem/1(phi), phi_ddot_numerator_subsystem/4(phi)
  FY/1 -> phi_ddot_numerator_subsystem/1(FY)
  theta_dot/1 -> phi_ddot_numerator_subsystem/5(theta_dot)
  phi_dot/1 -> phi_ddot_numerator_subsystem/3(phi_dot)
  theta/1 -> phi_ddot_numerator_subsystem/6(theta), phi_ddot_denominator_subsystem/2(theta)
  psi_dot/1 -> phi_ddot_numerator_subsystem/2(psi_dot)
  Divide/1 -> phi_ddot/1
  phi_ddot_denominator_subsystem/1(phi_ddot_denominator) -> Divide/2
  Ixx/1 -> phi_ddot_denominator_subsystem/3(Ixx)
  Iyy/1 -> phi_ddot_denominator_subsystem/4(Iyy), phi_ddot_numerator_subsystem/7(Iyy)
  Izz/1 -> phi_ddot_numerator_subsystem/8(Izz), phi_ddot_denominator_subsystem/5(Izz)
  K_phi/1 -> phi_ddot_numerator_subsystem/9(K_phi)
  D_phi/1 -> phi_ddot_numerator_subsystem/10(D_phi)
  h/1 -> phi_ddot_numerator_subsystem/11(h)

== system ISController/Vehicle_Sim/Vehicle_model/psi_subsystem ==
  FX : Inport  OutDataTypeStr=double  SampleTime=Ts
  FY : Inport  Port=2  OutDataTypeStr=double  SampleTime=Ts
  MZ : Inport  Port=3  OutDataTypeStr=double  SampleTime=Ts
  phi : Inport  Port=4  OutDataTypeStr=double  SampleTime=Ts
  theta : Inport  Port=5  OutDataTypeStr=double  SampleTime=Ts
  Ixx : Inport  Port=6  OutDataTypeStr=double  SampleTime=Ts
  Iyy : Inport  Port=7  OutDataTypeStr=double  SampleTime=Ts
  Izz : Inport  Port=8  OutDataTypeStr=double  SampleTime=Ts
  h : Inport  Port=9  OutDataTypeStr=double  SampleTime=Ts
  Add : Sum
  Add1 : Sum  Inputs=+-
  Add2 : Sum
  Add3 : Sum
  Divide{,1..6,8} (8 alike) : Product  Inputs=**
  Divide7 : Product  Inputs=*/
  Square{,1..3} (4 alike) : Math  Operator=square  RndMeth=Zero  SaturateOnIntegerOverflow=on
  Trigonometric Function : Trigonometry
  Trigonometric Function1 : Trigonometry
  Trigonometric Function2 : Trigonometry  Operator=cos
  Trigonometric Function3 : Trigonometry  Operator=cos
  psi_ddot : Outport
  wires:
  Square/1 -> Divide3/1
  MZ/1 -> Add1/1
  Trigonometric Function2/1 -> Square2/1, Divide2/1
  Divide2/1 -> Add/2
  Ixx/1 -> Divide3/2
  Add2/1 -> Divide4/2
  Square2/1 -> Divide6/2
  Divide6/1 -> Add2/2
  Divide3/1 -> Add3/1
  Add3/1 -> Divide7/2
  FY/1 -> Divide1/1
  FX/1 -> Divide/1
  Trigonometric Function3/1 -> Square3/1
  Iyy/1 -> Divide5/1
  Divide1/1 -> Divide2/2
  Square3/1 -> Divide4/1
  Izz/1 -> Divide6/1
  Trigonometric Function/1 -> Square/1, Divide1/2
  Trigonometric Function1/1 -> Square1/1, Divide/2
  phi/1 -> Trigonometric Function1/1, Trigonometric Function2/1
  theta/1 -> Trigonometric Function3/1, Trigonometric Function/1
  Divide8/1 -> Add1/2
  Add/1 -> Divide8/1
  Divide5/1 -> Add2/1
  Add1/1 -> Divide7/1
  Divide/1 -> Add/1
  Divide7/1 -> psi_ddot/1  "psi_ddot"
  Divide4/1 -> Add3/2
  Square1/1 -> Divide5/2
  h/1 -> Divide8/2

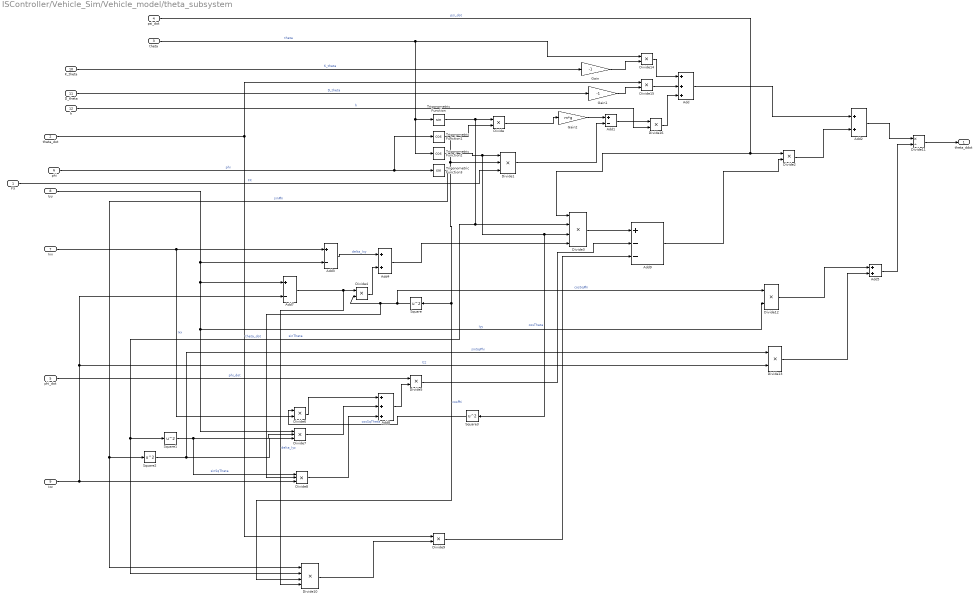
== system ISController/Vehicle_Sim/Vehicle_model/theta_subsystem ==
  FX : Inport  OutDataTypeStr=double  SampleTime=Ts
  theta_dot : Inport  Port=2  OutDataTypeStr=double  SampleTime=Ts
  theta : Inport  Port=3  OutDataTypeStr=double  SampleTime=Ts
  psi_dot : Inport  Port=4  OutDataTypeStr=double  SampleTime=Ts
  phi_dot : Inport  Port=5  OutDataTypeStr=double  SampleTime=Ts
  phi : Inport  Port=6  OutDataTypeStr=double  SampleTime=Ts
  Ixx : Inport  Port=7  OutDataTypeStr=double  SampleTime=Ts
  Iyy : Inport  Port=8  OutDataTypeStr=double  SampleTime=Ts
  Izz : Inport  Port=9  OutDataTypeStr=double  SampleTime=Ts
  K_theta : Inport  Port=10  OutDataTypeStr=double  SampleTime=Ts
  D_theta : Inport  Port=11  OutDataTypeStr=double  SampleTime=Ts
  h : Inport  Port=12  OutDataTypeStr=double  SampleTime=Ts
  Add : Sum  Inputs=+++
  Add1 : Sum  Inputs=+-
  Add2 : Sum
  Add3 : Sum  Inputs=+-
  Add4 : Sum
  Add5 : Sum
  Add7 : Sum  Inputs=+-
  Add8 : Sum  Inputs=+++
  Add9 : Sum  Inputs=+--
  Divide{,2,4..6,9,12..16} (11 alike) : Product  Inputs=**
  Divide1 : Product  Inputs=***
  Divide10 : Product  Inputs=****
  Divide11 : Product  Inputs=*/
  Divide3 : Product  Inputs=****
  Divide7 : Product  Inputs=***
  Divide8 : Product  Inputs=***
  Gain : Gain  Gain=-1  OutDataTypeStr=double
  Gain1 : Gain  Gain=-1  OutDataTypeStr=double
  Gain2 : Gain  Gain=m*g  OutDataTypeStr=double
  Square{,1..3} (4 alike) : Math  Operator=square  RndMeth=Zero  SaturateOnIntegerOverflow=on
  Trigonometric Function : Trigonometry
  Trigonometric Function1 : Trigonometry  Operator=cos
  Trigonometric Function2 : Trigonometry  Operator=cos
  Trigonometric Function3 : Trigonometry
  theta_ddot : Outport  OutDataTypeStr=double  SampleTime=Tsmall
  wires:
  Add/1 -> Add2/1
  Divide8/1 -> Add8/3
  Add4/1 -> Divide3/4
  Divide1/1 -> Add1/2
  Add8/1 -> Divide5/2
  Add1/1 -> Divide16/1
  Square1/1 -> Divide8/1, Divide7/2  "sinSqTheta"
  Divide7/1 -> Add8/2
  Add9/1 -> Divide2/2
  Square/1 -> Divide12/1, Divide8/2, Divide4/2  "cosSqPhi"
  Trigonometric Function3/1 -> Divide10/1, Square2/1  "sinPhi"
  Gain2/1 -> Add1/1
  Square2/1 -> Divide13/1, Divide7/3  "sinSqPhi"
  Trigonometric Function2/1 -> Square3/1, Divide3/3, Divide1/1  "cosTheta"
  Divide/1 -> Gain2/1
  Divide10/1 -> Divide9/2
  Trigonometric Function/1 -> Divide10/2, Square1/1, Divide3/2, Divide/1  "sinTheta"
  Divide6/1 -> Add8/1
  Divide2/1 -> Add2/2
  Divide9/1 -> Add9/3
  Divide5/1 -> Add9/2
  Gain/1 -> Divide14/2
  Divide4/1 -> Add4/2
  Add3/1 -> Add4/1  "delta_Ixy"
  Divide3/1 -> Add9/1
  Trigonometric Function1/1 -> Divide10/3, Square/1, Divide1/2, Divide/2  "cosPhi"
  Add7/1 -> Divide10/4, Divide4/1  "delta_Iyz"
  Divide16/1 -> Add/3
  Gain1/1 -> Divide15/2
  theta/1 -> Divide14/1, Trigonometric Function/1, Trigonometric Function2/1  "theta"
  Iyy/1 -> Divide7/1, Divide12/2, Add7/1, Add3/2  "Iyy"
  phi_dot/1 -> Divide5/1  "phi_dot"
  Ixx/1 -> Add3/1, Divide6/2  "Ixx"
  FX/1 -> Divide1/3  "FX"
  theta_dot/1 -> Divide15/1, Divide9/1  "theta_dot"
  Izz/1 -> Divide13/2, Add7/2, Divide8/3  "Izz"
  phi/1 -> Trigonometric Function1/1, Trigonometric Function3/1  "phi"
  psi_dot/1 -> Divide3/1, Divide2/1  "psi_dot"
  Add2/1 -> Divide11/1
  Divide11/1 -> theta_ddot/1
  Add5/1 -> Divide11/2
  Divide12/1 -> Add5/1
  Divide13/1 -> Add5/2
  Divide15/1 -> Add/2
  Divide14/1 -> Add/1
  K_theta/1 -> Gain/1  "K_theta"
  D_theta/1 -> Gain1/1  "D_theta"
  h/1 -> Divide16/2  "h"
  Square3/1 -> Divide6/1  "cosSqTheta"

== system ISController/Vehicle_Sim1/Vehicle_model/F_M_subsystem ==
  Fx1 : Inport  OutDataTypeStr=double  SampleTime=Ts
  Fx2 : Inport  Port=2  OutDataTypeStr=double  SampleTime=Ts
  Fx3 : Inport  Port=3  OutDataTypeStr=double  SampleTime=Ts
  Fx4 : Inport  Port=4  OutDataTypeStr=double  SampleTime=Ts
  Fy1 : Inport  Port=5  OutDataTypeStr=double  SampleTime=Ts
  Fy2 : Inport  Port=6  OutDataTypeStr=double  SampleTime=Ts
  Fy3 : Inport  Port=7  OutDataTypeStr=double  SampleTime=Ts
  Fy4 : Inport  Port=8  OutDataTypeStr=double  SampleTime=Ts
  l_f : Inport  Port=9  OutDataTypeStr=double  SampleTime=Ts
  l_r : Inport  Port=10  OutDataTypeStr=double  SampleTime=Ts
  w : Inport  Port=11  OutDataTypeStr=double  SampleTime=Ts
  Add : Sum  Inputs=++++
  Add1 : Sum  Inputs=++++
  Add2 : Sum  Inputs=++--
  Add3 : Sum
  Add4 : Sum
  Product{,1..3} (4 alike) : Product
  Subtract : Sum  Inputs=+-
  Subtract1 : Sum
  FX : Outport
  FY : Outport  Port=2
  Mz : Outport  Port=3
  wires:
  Fy2/1 -> Add3/2, Add1/2  "Fy2"
  Fx3/1 -> Subtract1/1, Add/1
  Fx4/1 -> Subtract1/2, Add/2
  Fx1/1 -> Subtract/2, Add/3  "Fx1"
  Fx2/1 -> Subtract/1, Add/4  "Fx2"
  Add/1 -> FX/1
  Fy1/1 -> Add3/1, Add1/1  "Fy1"
  Fy3/1 -> Add4/1, Add1/3
  Fy4/1 -> Add4/2, Add1/4
  Add1/1 -> FY/1
  Add2/1 -> Mz/1
  Add3/1 -> Product/1
  l_f/1 -> Product/2
  Product/1 -> Add2/1
  Subtract/1 -> Product1/2
  w/1 -> Product3/2, Product1/1
  Product1/1 -> Add2/2
  Add4/1 -> Product2/1
  l_r/1 -> Product2/2
  Product2/1 -> Add2/3
  Subtract1/1 -> Product3/1
  Product3/1 -> Add2/4

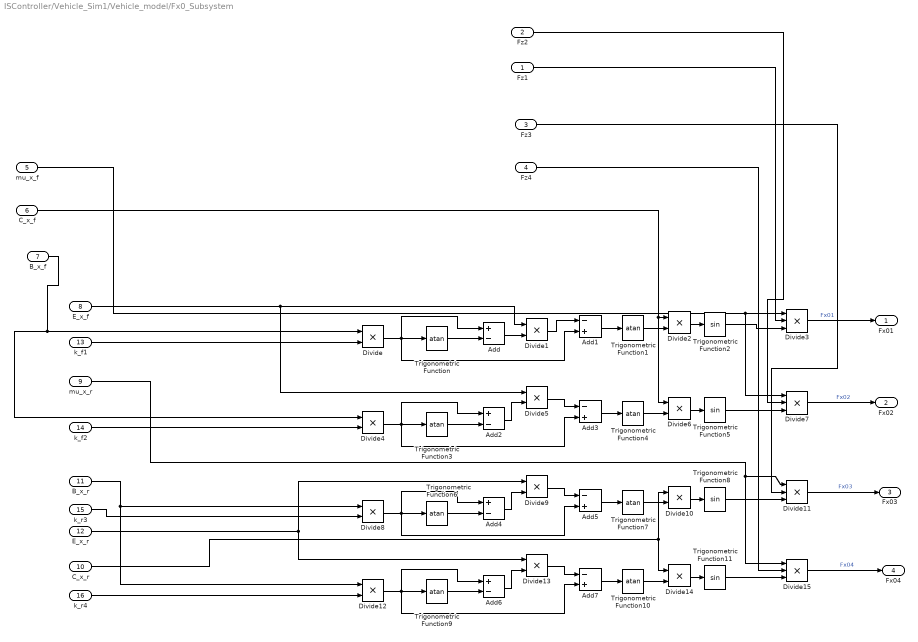
== system ISController/Vehicle_Sim1/Vehicle_model/Fx0_Subsystem ==
  Fz1 : Inport  OutDataTypeStr=double  SampleTime=Ts
  Fz2 : Inport  Port=2  OutDataTypeStr=double  SampleTime=Ts
  Fz3 : Inport  Port=3  OutDataTypeStr=double  SampleTime=Ts
  Fz4 : Inport  Port=4  OutDataTypeStr=double  SampleTime=Ts
  mu_x_f : Inport  Port=5
  C_x_f : Inport  Port=6
  B_x_f : Inport  Port=7
  E_x_f : Inport  Port=8
  mu_x_r : Inport  Port=9
  C_x_r : Inport  Port=10
  B_x_r : Inport  Port=11
  E_x_r : Inport  Port=12
  k_f1 : Inport  Port=13
  k_f2 : Inport  Port=14
  k_r3 : Inport  Port=15
  k_r4 : Inport  Port=16
  Add{,2,4,6} (4 alike) : Sum  Inputs=+-
  Add{1,3,5,7} (4 alike) : Sum  Inputs=-+
  Divide{,1..2,4..6,8..10,12..14} (12 alike) : Product  Inputs=**
  Divide{3,7,11,15} (4 alike) : Product  Inputs=***
  Trigonometric Function{,1,3..4,6..7,9..10} (8 alike) : Trigonometry  Operator=atan
  Trigonometric Function{2,5,8,11} (4 alike) : Trigonometry
  Fx01 : Outport  OutDataTypeStr=double  SampleTime=Ts
  Fx02 : Outport  Port=2  OutDataTypeStr=double  SampleTime=Ts
  Fx03 : Outport  Port=3  OutDataTypeStr=double  SampleTime=Ts
  Fx04 : Outport  Port=4  OutDataTypeStr=double  SampleTime=Ts
  wires:
  Divide13/1 -> Add7/1
  Trigonometric Function2/1 -> Divide3/3
  Divide11/1 -> Fx03/1  "Fx03"
  Divide7/1 -> Fx02/1  "Fx02"
  Divide1/1 -> Add1/1
  Trigonometric Function/1 -> Add/2
  Divide15/1 -> Fx04/1  "Fx04"
  Add/1 -> Divide1/2
  Divide/1 -> Add1/2, Add/1, Trigonometric Function/1
  k_f1/1 -> Divide/2
  k_r4/1 -> Divide12/2
  k_r3/1 -> Divide8/2
  Divide6/1 -> Trigonometric Function5/1
  Divide4/1 -> Add3/2, Add2/1, Trigonometric Function3/1
  Divide5/1 -> Add3/1
  Trigonometric Function3/1 -> Add2/2
  Add2/1 -> Divide5/2
  E_x_f/1 -> Divide5/1, Divide1/1
  B_x_f/1 -> Divide4/1, Divide/1
  Trigonometric Function4/1 -> Divide6/2
  C_x_f/1 -> Divide6/1, Divide2/1
  Trigonometric Function5/1 -> Divide7/3
  Add3/1 -> Trigonometric Function4/1
  C_x_r/1 -> Divide14/1, Divide10/1
  B_x_r/1 -> Divide12/1, Divide8/1
  E_x_r/1 -> Divide9/1, Divide13/1
  mu_x_r/1 -> Divide15/1, Divide11/1
  Fz2/1 -> Divide7/2
  mu_x_f/1 -> Divide7/1, Divide3/1
  k_f2/1 -> Divide4/2
  Fz1/1 -> Divide3/2
  Fz3/1 -> Divide11/2
  Add1/1 -> Trigonometric Function1/1
  Add4/1 -> Divide9/2
  Divide8/1 -> Add5/2, Add4/1, Trigonometric Function6/1
  Trigonometric Function8/1 -> Divide11/3
  Add5/1 -> Trigonometric Function7/1
  Trigonometric Function6/1 -> Add4/2
  Divide10/1 -> Trigonometric Function8/1
  Trigonometric Function7/1 -> Divide10/2
  Fz4/1 -> Divide15/2
  Divide9/1 -> Add5/1
  Trigonometric Function1/1 -> Divide2/2
  Divide3/1 -> Fx01/1  "Fx01"
  Divide2/1 -> Trigonometric Function2/1
  Trigonometric Function10/1 -> Divide14/2
  Trigonometric Function9/1 -> Add6/2
  Divide14/1 -> Trigonometric Function11/1
  Divide12/1 -> Add7/2, Add6/1, Trigonometric Function9/1
  Trigonometric Function11/1 -> Divide15/3
  Add7/1 -> Trigonometric Function10/1
  Add6/1 -> Divide13/2

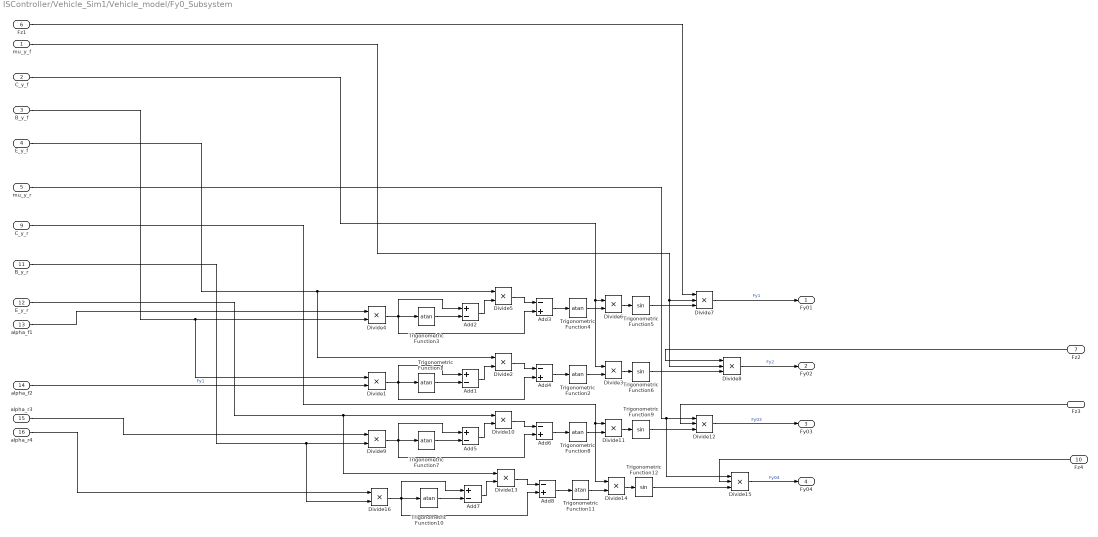
== system ISController/Vehicle_Sim1/Vehicle_model/Fy0_Subsystem ==
  mu_y_f : Inport  OutDataTypeStr=double  SampleTime=Ts
  C_y_f : Inport  Port=2  OutDataTypeStr=double  SampleTime=Ts
  B_y_f : Inport  Port=3  OutDataTypeStr=double  SampleTime=Ts
  E_y_f : Inport  Port=4  OutDataTypeStr=double  SampleTime=Ts
  mu_y_r : Inport  Port=5  OutDataTypeStr=double  SampleTime=Ts
  Fz1 : Inport  Port=6  OutDataTypeStr=double  SampleTime=Ts
  Fz2 : Inport  Port=7  OutDataTypeStr=double  SampleTime=Ts
  Fz3 : Inport  Port=8  OutDataTypeStr=double  SampleTime=Ts
  C_y_r : Inport  Port=9  OutDataTypeStr=double  SampleTime=Ts
  Fz4 : Inport  Port=10  OutDataTypeStr=double  SampleTime=Ts
  B_y_r : Inport  Port=11  OutDataTypeStr=double  SampleTime=Ts
  E_y_r : Inport  Port=12  OutDataTypeStr=double  SampleTime=Ts
  alpha_f1 : Inport  Port=13  OutDataTypeStr=double  SampleTime=Ts
  alpha_f2 : Inport  Port=14  OutDataTypeStr=double  SampleTime=Ts
  alpha_r3 : Inport  Port=15  OutDataTypeStr=double  SampleTime=Ts
  alpha_r4 : Inport  Port=16  OutDataTypeStr=double  SampleTime=Ts
  Add{1..2,5,7} (4 alike) : Sum  Inputs=+-
  Add{3..4,6,8} (4 alike) : Sum  Inputs=-+
  Divide{1..6,9..11,13..14,16} (12 alike) : Product  Inputs=**
  Divide{7..8,12,15} (4 alike) : Product  Inputs=***
  Trigonometric Function{1..4,7..8,10..11} (8 alike) : Trigonometry  Operator=atan
  Trigonometric Function{5..6,9,12} (4 alike) : Trigonometry
  Fy01 : Outport  OutDataTypeStr=double  SampleTime=Ts
  Fy02 : Outport  Port=2  OutDataTypeStr=double  SampleTime=Ts
  Fy03 : Outport  Port=3  OutDataTypeStr=double  SampleTime=Ts
  Fy04 : Outport  Port=4  OutDataTypeStr=double  SampleTime=Ts
  wires:
  Add6/1 -> Trigonometric Function8/1
  Trigonometric Function9/1 -> Divide12/3
  alpha_r3/1 -> Divide9/1
  alpha_r4/1 -> Divide16/1
  C_y_f/1 -> Divide6/1, Divide3/1
  B_y_f/1 -> Divide4/2, Divide1/1
  alpha_f1/1 -> Divide4/1
  E_y_r/1 -> Divide13/1, Divide10/1
  B_y_r/1 -> Divide16/2, Divide9/2
  mu_y_r/1 -> Divide12/1, Divide15/1
  E_y_f/1 -> Divide5/1, Divide2/1
  mu_y_f/1 -> Divide8/2, Divide7/2
  Trigonometric Function1/1 -> Add1/2
  Add1/1 -> Divide2/2
  Trigonometric Function6/1 -> Divide8/3
  Trigonometric Function2/1 -> Divide3/2
  Divide1/1 -> Add4/2, Add1/1, Trigonometric Function1/1
  Divide3/1 -> Trigonometric Function6/1
  Divide2/1 -> Add4/1
  Add4/1 -> Trigonometric Function2/1
  Fz4/1 -> Divide15/2
  Fz3/1 -> Divide12/2
  Fz2/1 -> Divide8/1
  Fz1/1 -> Divide7/1
  C_y_r/1 -> Divide14/1, Divide11/1
  Divide15/1 -> Fy04/1  "Fy04"
  Trigonometric Function12/1 -> Divide15/3
  Add8/1 -> Trigonometric Function11/1
  Divide16/1 -> Add8/2, Add7/1, Trigonometric Function10/1
  Trigonometric Function11/1 -> Divide14/2
  Add7/1 -> Divide13/2
  Divide13/1 -> Add8/1
  Divide14/1 -> Trigonometric Function12/1
  Trigonometric Function10/1 -> Add7/2
  Divide12/1 -> Fy03/1  "Fy03"
  Divide9/1 -> Add6/2, Add5/1, Trigonometric Function7/1
  Trigonometric Function7/1 -> Add5/2
  Add5/1 -> Divide10/2
  Trigonometric Function5/1 -> Divide7/3
  Divide11/1 -> Trigonometric Function9/1
  Divide6/1 -> Trigonometric Function5/1
  Add3/1 -> Trigonometric Function4/1
  Trigonometric Function3/1 -> Add2/2
  Divide10/1 -> Add6/1
  Add2/1 -> Divide5/2
  Trigonometric Function4/1 -> Divide6/2
  Divide4/1 -> Add3/2, Add2/1, Trigonometric Function3/1
  Divide5/1 -> Add3/1
  Trigonometric Function8/1 -> Divide11/2
  Divide7/1 -> Fy01/1  "Fy1"
  Divide8/1 -> Fy02/1  "Fy2"
  alpha_f2/1 -> Divide1/2  "Fy1"

== system ISController/Vehicle_Sim1/Vehicle_model/Fy0_to_Fy_subsystem ==
  mu_x_f : Inport  OutDataTypeStr=double  SampleTime=Ts
  mu_x_r : Inport  Port=2  OutDataTypeStr=double  SampleTime=Ts
  Fx01 : Inport  Port=3  OutDataTypeStr=double  SampleTime=Ts
  Fx02 : Inport  Port=4  OutDataTypeStr=double  SampleTime=Ts
  Fx03 : Inport  Port=5  OutDataTypeStr=double  SampleTime=Ts
  Fx04 : Inport  Port=6  OutDataTypeStr=double  SampleTime=Ts
  Fz1 : Inport  Port=7  OutDataTypeStr=double  SampleTime=Ts
  Fz2 : Inport  Port=8  OutDataTypeStr=double  SampleTime=Ts
  Fz3 : Inport  Port=9  OutDataTypeStr=double  SampleTime=Ts
  Fz4 : Inport  Port=10  OutDataTypeStr=double  SampleTime=Ts
  Fy01 : Inport  Port=11  OutDataTypeStr=double  SampleTime=Ts
  Fy02 : Inport  Port=12  OutDataTypeStr=double  SampleTime=Ts
  Fy03 : Inport  Port=13  OutDataTypeStr=double  SampleTime=Ts
  Fy04 : Inport  Port=14  OutDataTypeStr=double  SampleTime=Ts
  Add{,1..3} (4 alike) : Sum  Inputs=+-
  Constant{,1..3} (4 alike) : Constant
  Divide{,3,6,9} (4 alike) : Product  Inputs=*/
  Divide{1..2,4..5,7..8,10..11} (8 alike) : Product  Inputs=**
  Sqrt{,1..3} (4 alike) : Sqrt  SaturateOnIntegerOverflow=on
  Square{,1..3} (4 alike) : Math  Operator=square  RndMeth=Zero  SaturateOnIntegerOverflow=on
  local_Fy1 : Outport  OutDataTypeStr=double  SampleTime=Ts
  local_Fy2 : Outport  Port=2  OutDataTypeStr=double  SampleTime=Ts
  local_Fy3 : Outport  Port=3  OutDataTypeStr=double  SampleTime=Ts
  lcoal_Fy4 : Outport  Port=4  OutDataTypeStr=double  SampleTime=Ts
  wires:
  Divide1/1 -> Divide/2
  Divide/1 -> Square/1
  Constant/1 -> Add/1
  Divide2/1 -> local_Fy1/1  "Fy1"
  Divide11/1 -> lcoal_Fy4/1  "Fy4"
  Fz4/1 -> Divide10/2  "Fz4"
  mu_x_f/1 -> Divide4/1, Divide1/1  "mu_x_f"
  Fx04/1 -> Divide9/1  "Fx04"
  Fx01/1 -> Divide/1  "Fx01"
  Fz3/1 -> Divide7/2  "Fz3"
  Fx02/1 -> Divide3/1  "Fx02"
  mu_x_r/1 -> Divide10/1, Divide7/1  "mu_x_r"
  Fx03/1 -> Divide6/1  "Fx03"
  Fz1/1 -> Divide1/2  "Fz1"
  Fz2/1 -> Divide4/2  "Fz2"
  Square2/1 -> Add2/2
  Divide6/1 -> Square2/1
  Sqrt2/1 -> Divide8/1
  Constant2/1 -> Add2/1
  Sqrt3/1 -> Divide11/1
  Constant3/1 -> Add3/1
  Add3/1 -> Sqrt3/1
  Divide9/1 -> Square3/1
  Square3/1 -> Add3/2
  Add/1 -> Sqrt/1
  Square/1 -> Add/2
  Divide10/1 -> Divide9/2
  Divide8/1 -> local_Fy3/1  "Fy3"
  Sqrt/1 -> Divide2/1
  Divide4/1 -> Divide3/2
  Square1/1 -> Add1/2
  Divide3/1 -> Square1/1
  Constant1/1 -> Add1/1
  Fy02/1 -> Divide5/2  "Fy02"
  Add1/1 -> Sqrt1/1
  Sqrt1/1 -> Divide5/1
  Divide7/1 -> Divide6/2
  Add2/1 -> Sqrt2/1
  Fy03/1 -> Divide8/2  "Fy03"
  Divide5/1 -> local_Fy2/1  "Fy2"
  Fy01/1 -> Divide2/2  "Fy01"
  Fy04/1 -> Divide11/2  "Fy04"
